simulink model "aMedianFilter_forC"  (Simulink 7.7)
settings: Solver=FixedStepDiscrete  SolverMode=SingleTasking  StartTime=0.0  StopTime=131*131  FixedStep=1  RelTol=1e-3
InitFcn:
  | wsize1 = uint32(3);
  | wsize2 = uint32(5);
  | wsize3 = uint32(7);
undefined symbols (not defined in the file): jet
libraries: vipsnks x2, vipsrcs x1
settings Model: Creator=kkintali  LastModifiedBy=kkintali  ExtModeAutoUpdateStatusClock=off
settings DataIOCC: SaveOutput=off  SignalLogging=off  SaveTime=off
settings OptimizationCC: BlockReduction=off  ConditionallyExecuteInputs=off  InlineParams=on  InitFltsAndDblsToZero=on  EfficientMapNaN2IntZero=off
settings DebuggingCC: AlgebraicLoopMsg=error  SingleTaskRateTransMsg=error  StrictBusMsg=Warning
settings HardwareCC: ProdHWDeviceType=ASIC/FPGA->ASIC/FPGA
settings SFSimCC: SimParseCustomCode=off

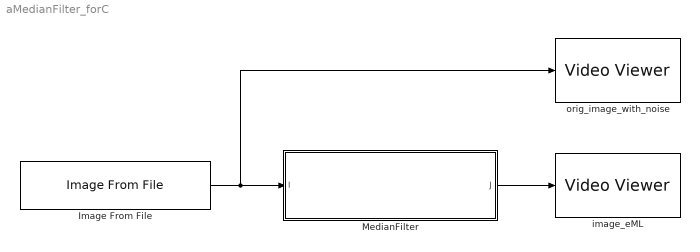
== system aMedianFilter_forC ==
  Image From File : vipsrcs/Image From File  Tag=vipblks_nd  SystemSampleTime=-1  FileName=pattern_noisy_002.tif  imagePorts=One multidimensional signal  Ts=131*131  ImageDataType=uint8  Signed=on  WordLength=16  sdImageDataType=uint(8)  FractionLengthMode=User-defined  FractionLength=15  OutPortLabels=R
  MedianFilter : Stateflow chart  TreatAsAtomicUnit=on
  image_eML : vipsnks/Video Viewer  inputType=Obsolete7b  imagePorts=One multidimensional signal  useColorMap=off  colormapValue=jet(256);  specRange=off  minInputVal=0  maxInputVal=255  FigPos=[998 1155 237 176]  AxisZoom=on  trueSizedOnce=on  OpenAtMdlStart=on
  orig_image_with_noise : vipsnks/Video Viewer  inputType=Obsolete7b  imagePorts=One multidimensional signal  useColorMap=off  colormapValue=jet(256);  specRange=off  minInputVal=0  maxInputVal=255  FigPos=[725 1157 253 176]  AxisZoom=on  trueSizedOnce=on  OpenAtMdlStart=on
  wires:
  Image From File/1 -> orig_image_with_noise/1, MedianFilter/1(I)
  MedianFilter/1(J) -> image_eML/1

== matlab function MedianFilter ==
  data: I input double; J output double
function J = amedfilt2_calc(I)

J = amedfilt2_calc(I);
